simulink model "Copy_of_modelo8_simulink_controle_integral_doc"  (R2023b)
settings: Solver=VariableStepAuto  StartTime=0.0  StopTime=25  RelTol=1e-3
undefined symbols (not defined in the file or in its folder): Ar, Br, C_psi, Cr, F_psi, G_psi, Ki, Kx
settings Model: Creator=Talles  LastModifiedBy=Talles
settings DataIOCC: SaveFormat=Array  Refine=10

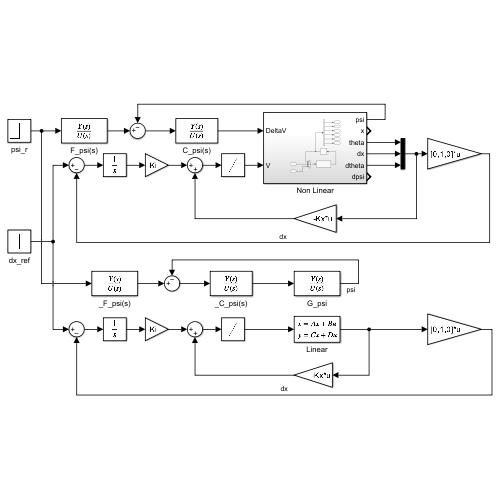
[thumbnail: Simulink's stored preview of the top-level diagram]
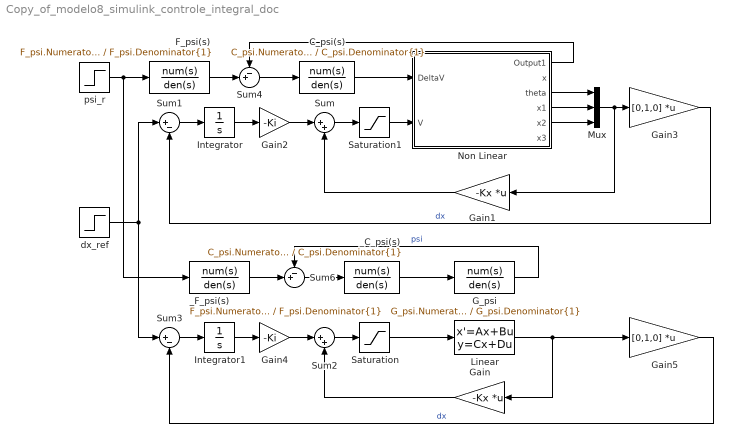
== system Copy_of_modelo8_simulink_controle_integral_doc ==
  C_psi(s) : TransferFcn  Numerator=C_psi.Numerator{1}  Denominator=C_psi.Denominator{1}
  F_psi(s) : TransferFcn  Numerator=F_psi.Numerator{1}  Denominator=F_psi.Denominator{1}
  G_psi : TransferFcn  Numerator=G_psi.Numerator{1}  Denominator=G_psi.Denominator{1}
  Gain : Gain  Gain=-Kx  Multiplication=Matrix(K*u)
  Gain1 : Gain  Gain=-Kx  Multiplication=Matrix(K*u)
  Gain2 : Gain  Gain=-Ki
  Gain3 : Gain  Gain=[0,1,0]  Multiplication=Matrix(K*u)
  Gain4 : Gain  Gain=-Ki
  Gain5 : Gain  Gain=[0,1,0]  Multiplication=Matrix(K*u)
  Integrator : Integrator
  Integrator1 : Integrator
  Linear : StateSpace  A=Ar  B=Br  C=Cr  D=zeros(3,1)  InitialCondition=zeros(3,1)
  Mux : Mux  Inputs=3
  Non Linear : Subsystem
  Saturation : Saturate  UpperLimit=7.4  LowerLimit=-7.4
  Saturation1 : Saturate  UpperLimit=7.4  LowerLimit=-7.4
  Sum : Sum  Inputs=|++
  Sum1 : Sum  Inputs=|+-
  Sum2 : Sum  Inputs=|++
  Sum3 : Sum  Inputs=|+-
  Sum4 : Sum  Inputs=-+|
  Sum6 : Sum  Inputs=-+|
  _C_psi(s) : TransferFcn  Numerator=C_psi.Numerator{1}  Denominator=C_psi.Denominator{1}
  _F_psi(s) : TransferFcn  Numerator=F_psi.Numerator{1}  Denominator=F_psi.Denominator{1}
  dx_ref : Step  Time=10  After=0.3  SampleTime=0
  psi_r : Step  Time=15  After=pi/2  SampleTime=0
  wires:
  Linear/1 -> Gain5/1, Gain/1
  Saturation/1 -> Linear/1
  Non Linear/3(theta) -> Mux/1
  Non Linear/4(x1) -> Mux/2
  Gain1/1 -> Sum/2
  Saturation1/1 -> Non Linear/2(V)
  Non Linear/5(x2) -> Mux/3
  Mux/1 -> Gain3/1, Gain1/1
  Sum/1 -> Saturation1/1
  Integrator/1 -> Gain2/1
  Gain2/1 -> Sum/1
  Sum1/1 -> Integrator/1
  dx_ref/1 -> Sum3/1, Sum1/1
  Sum3/1 -> Integrator1/1
  Gain4/1 -> Sum2/1
  Integrator1/1 -> Gain4/1
  Sum2/1 -> Saturation/1
  Gain/1 -> Sum2/2
  Gain5/1 -> Sum3/2  "dx"
  C_psi(s)/1 -> Non Linear/1(DeltaV)
  Sum4/1 -> C_psi(s)/1
  F_psi(s)/1 -> Sum4/2
  Non Linear/1(Output1) -> Sum4/1
  Gain3/1 -> Sum1/2  "dx"
  psi_r/1 -> F_psi(s)/1, _F_psi(s)/1
  _F_psi(s)/1 -> Sum6/2
  Sum6/1 -> _C_psi(s)/1
  _C_psi(s)/1 -> G_psi/1
  G_psi/1 -> Sum6/1  "psi"

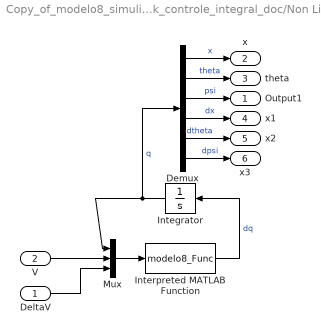
== system Copy_of_modelo8_simulink_controle_integral_doc/Non Linear ==
  DeltaV : Inport
  V : Inport  Port=2
  Demux : Demux  Outputs=6
  Integrator : Integrator  InitialCondition=[0;0;0;0;0;0]
  Interpreted MATLAB Function : MATLABFcn  MATLABFcn=modelo8_Func  OutputDimensions=6  OutputSignalType=real
  Mux : Mux  Inputs=3
  Output1 : Outport
  x : Outport  Port=2
  theta : Outport  Port=3
  x1 : Outport  Port=4
  x2 : Outport  Port=5
  x3 : Outport  Port=6
  wires:
  Interpreted MATLAB Function/1 -> Integrator/1  "dq"
  Integrator/1 -> Demux/1, Mux/1  "q"
  Demux/3 -> Output1/1  "psi"
  Mux/1 -> Interpreted MATLAB Function/1
  Demux/1 -> x/1  "x"
  Demux/2 -> theta/1  "theta"
  V/1 -> Mux/2
  Demux/4 -> x1/1  "dx"
  Demux/5 -> x2/1  "dtheta"
  Demux/6 -> x3/1  "dpsi"
  DeltaV/1 -> Mux/3
